simulink model "Maglev_SSC_ideal"  (R2025a)
settings: Solver=ode23t  StartTime=0.0  StopTime=T_sim  FixedStep=0.01  RelTol=1e-3  AbsTol=1e-3
PreLoadFcn:
  | modelPath = fileparts(which(bdroot));
  | run(fullfile(fileparts(modelPath), 'setup_sim_params.m'));
  | load(fullfile(fileparts(modelPath), 'Controller_Params', 'EKFData.mat'));
  | load(fullfile(fileparts(modelPath), 'Controller_Params', 'LinearControllerData.mat'));
undefined symbols (not defined in the file): Ext_Fina_Val, Ext_Init_Val, grav, I_max, I_min, mass, Plant, SSC, T_stp
libraries: fl_lib x11, nesl_utility x4
settings Model: Creator=Meng Lingbing  LastModifiedBy=CelestialAurora
settings SolverCC: AutoScaleAbsTol=off  AlgebraicLoopSolver=TrustRegion  MaxZcPerStep=1.0
settings DebuggingCC: AlgebraicLoopMsg=none  UnconnectedInputMsg=warning  UnconnectedOutputMsg=warning  UnconnectedLineMsg=warning  SymbolicDimsDataTypeCodeGenerationDiagnostic=none
settings ModelReferenceCC: EnableRefExpFcnMdlSchedulingChecks=on
settings SFSimCC: CustomCodeUndefinedFunction=UseInterfaceOnly
settings RTWCC: GPUComputeCapability=3.5  DLArmComputeVersion=19.05
settings SimscapeCC: SimscapeLogType=all  SimscapeLogSimulationStatistics=on  SimscapeLogDataHistory=10000.0

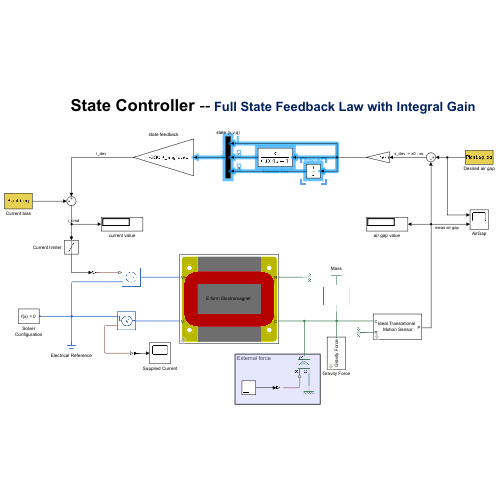
[thumbnail: Simulink's stored preview of the top-level diagram]
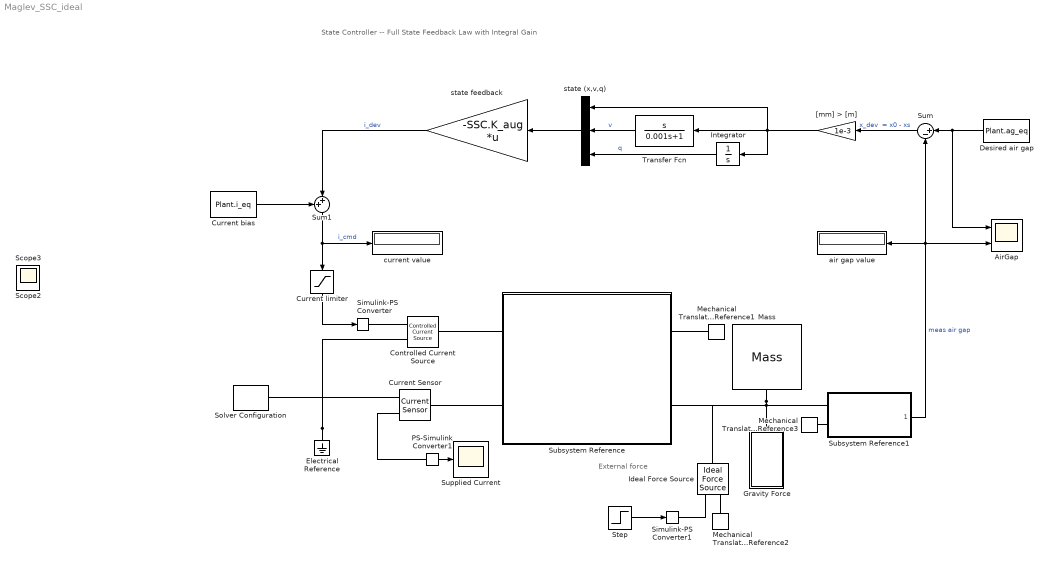
== system Maglev_SSC_ideal ==
  note: State Controller -- Full State Feedback Law with Integral Gain
  note: External force
  AirGap : Scope  NumInputPorts=2
      settings: ActiveDisplayYMinimum=0.98163587545275477  ActiveDisplayYMaximum=2.6687071249496941
  Controlled Current Source : fl_lib/Electrical/Electrical Sources/Controlled Current Source
  Current Sensor : fl_lib/Electrical/Electrical Sensors/Current Sensor
  Current bias : Constant  Value=Plant.i_eq
  Current limiter : Saturate  UpperLimit=I_max  LowerLimit=I_min
  Desired air gap : Constant  Value=Plant.ag_eq
  Electrical Reference : fl_lib/Electrical/Electrical Elements/Electrical Reference
  Gravity Force : Subsystem
      mask DialogControl DescGroupVar Prompt: Gravity Force
      mask DialogControl DescTextVar Prompt: Fg = Mass*grav, as constant parameters predefined
      mask DialogControl DescTextVar2 Prompt: Direction: Downward
      mask Display: disp("Gravity Force")
  Ideal Force Source : fl_lib/Mechanical/Mechanical Sources/Ideal Force Source
  Integrator : Integrator
  Mass : fl_lib/Mechanical/Translational Elements/Mass  mass=mass kg  num_ports=foundation.enum.numPorts2.one  v_specify=on  v_priority=Low  v=0 m/s  v_nominal_specify=off  v_nominal_value=1  v_nominal_unit=m/s  f_specify=off  f_priority=None  f=0 N  f_nominal_specify=off  f_nominal_value=700  f_nominal_unit=N
  Mechanical Translational Reference1 : fl_lib/Mechanical/Translational Elements/Mechanical Translational Reference
  Mechanical Translational Reference2 : fl_lib/Mechanical/Translational Elements/Mechanical Translational Reference
  Mechanical Translational Reference3 : fl_lib/Mechanical/Translational Elements/Mechanical Translational Reference
  PS-Simulink Converter1 : nesl_utility/PS-Simulink Converter  PhysicalDomain=network_engine_domain  SubClassName=ps_output  LeftPortType=input  RightPortType=output  PseudoPeriodic=off  Frequencies=[]  VectorFormat=inherit  Unit=inherit  AffineConversion=off
  Simulink-PS Converter : nesl_utility/Simulink-PS Converter  PhysicalDomain=network_engine_domain  SubClassName=ps_input  LeftPortType=input  RightPortType=output  PseudoPeriodic=off  Frequencies=[]  NoiseDistribution=none  NoiseParameters=[]  Unit=1  AffineConversion=off  FilteringAndDerivatives=zero  SimscapeFilterOrder=1  InputFilterTimeConstant=0.001  UdotUserProvided=0
  Simulink-PS Converter1 : nesl_utility/Simulink-PS Converter  PhysicalDomain=network_engine_domain  SubClassName=ps_input  LeftPortType=input  RightPortType=output  PseudoPeriodic=off  Frequencies=[]  NoiseDistribution=none  NoiseParameters=[]  Unit=1  AffineConversion=off  FilteringAndDerivatives=provide  SimscapeFilterOrder=1  InputFilterTimeConstant=0.001  UdotUserProvided=0
  Solver Configuration : nesl_utility/Solver Configuration  PhysicalDomain=network_engine_domain  SubClassName=solver  LeftPortType=input  RightPortType=generic  Tones=[]  Harmonics=[]  SimulateNoise=off  Profile=off  UseLocalSampling=off  EnableSwitchedLinearOptims=on  FrequencyDomain=off  UseCCode=off  RelTol=0.001  AbsTol=1e-06  MinStep=1e-09  ToWorkspace=off  RevertToSquareIcSolve=off  NumHomotopyIterations=100  PhasorMode=off  PhasorModeNumHarmonics=1  ConsistencySolver=NEWTON_XTOL_AFTER_FTOL  IndexReductionMethod=DerivativeReplacement  DoDC=off  ResidualTolerance=1e-09  ConsistencyTolSource=GLOBAL  ConsistencyAbsTol=0.001  ConsistencyRelTol=0.001  ConsistencyTolFactor=0.001  UseLocalSolver=off  LocalSolverChoice=NE_BACKWARD_EULER_ADVANCER  ResolveIndetEquations=on  FunctionEvalNumThread=1  LocalSolverSampleTime=0.001  DoFixedCost=off  MaxNonlinIter=3  MaxModeIter=2  ComputeImpulses=off  ImpulseIterations=2  LinearAlgebra=auto  LinearAlgebraNumThread=0  EquationFormulation=NE_TIME_EF  DelaysMemoryBudget=1024  AutomaticFiltering=on  FilteringTimeConstant=0.001  PartitionStorageMethod=AS_NEEDED  PartitionMemoryBudget=1024  PartitionMethod=ROBUST  MultibodyUseLocalSolver=off  MultibodyLocalSolverChoice=ODE1  MultibodyLocalSolverSampleTime=0.001
  Step : Step  Time=T_stp  Before=Ext_Init_Val  After=Ext_Fina_Val  SampleTime=0
  Subsystem Reference : Subsystem  ReferencedSubsystem=IntegratedElectromagnet  l_airgap=airgap_init
  Subsystem Reference1 : Subsystem  ReferencedSubsystem=IdealTrans_MotionSensor  ns_sw=isNoiseActive  ns_pw=NoisePower  ts=Ts  init_pos=airgap_init
  Sum : Sum  Inputs=|+-
  Sum1 : Sum  Inputs=++|
  Supplied Current : Scope
      settings: ActiveDisplayYMinimum=-2.195516974935928  ActiveDisplayYMaximum=17.297943585945966  DataLoggingVariableName=ScopeData3
  Transfer Fcn : TransferFcn  Numerator=[1 0]  Denominator=[0.001 1]
  "[mm] > [m]" : Gain  Gain=1e-3
  air gap value : Display
      settings: Decimation=4
  current value : Display
  state (x,v,q) : Mux  Inputs=3
  state feedback : Gain  Gain=-SSC.K_aug  Multiplication=Matrix(K*u) (u vector)
  Scope2 : Scope
      settings: ActiveDisplayYMinimum=2.68786  ActiveDisplayYMaximum=51.73117
  Scope3 : Scope
      settings: ActiveDisplayYMinimum=-19475.53313  ActiveDisplayYMaximum=27959.62036  DataLoggingVariableName=ScopeData2
  wires:
  state feedback/1 -> Sum1/2  "i_dev"
  Sum/1 -> "[mm] > [m]"/1  "x_dev  = x0 - xs"
  Subsystem Reference1/1 -> air gap value/1, AirGap/2, Sum/2  "meas air gap"
  Sum1/1 -> Current limiter/1, current value/1  "i_cmd"
  Desired air gap/1 -> Sum/1, AirGap/1
  Current limiter/1 -> Simulink-PS Converter/1
  Current bias/1 -> Sum1/1
  PS-Simulink Converter1/1 -> Supplied Current/1
  Integrator/1 -> state (x,v,q)/3  "q"
  state (x,v,q)/1 -> state feedback/1
  Transfer Fcn/1 -> state (x,v,q)/2  "v"
  Step/1 -> Simulink-PS Converter1/1
  "[mm] > [m]"/1 -> Transfer Fcn/1, state (x,v,q)/1, Integrator/1
  connections:
  Electrical Reference/LConn1 -- Solver Configuration/RConn1 -- Controlled Current Source/RConn2 -- Current Sensor/RConn2
  Mass/LConn1 -- Subsystem Reference1/LConn1 -- Gravity Force/RConn1 -- Subsystem Reference/RConn2 -- Ideal Force Source/LConn1
  Subsystem Reference/RConn1 -- Mechanical Translational Reference1/LConn1
  Simulink-PS Converter/RConn1 -- Controlled Current Source/RConn1
  Subsystem Reference/LConn2 -- Current Sensor/LConn1
  PS-Simulink Converter1/LConn1 -- Current Sensor/RConn1
  Subsystem Reference/LConn1 -- Controlled Current Source/LConn1
  Simulink-PS Converter1/RConn1 -- Ideal Force Source/RConn1
  Mechanical Translational Reference2/LConn1 -- Ideal Force Source/RConn2
  Mechanical Translational Reference3/LConn1 -- Subsystem Reference1/LConn2

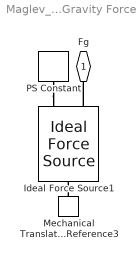
== system Maglev_SSC_ideal/Gravity Force ==
  Ideal Force Source1 : fl_lib/Mechanical/Mechanical Sources/Ideal Force Source
  Mechanical Translational Reference3 : fl_lib/Mechanical/Translational Elements/Mechanical Translational Reference
  PS Constant : fl_lib/Physical Signals/Sources/PS Constant  constant=mass*grav N
  Fg : PMIOPort  Side=Right
  connections:
  Mechanical Translational Reference3/LConn1 -- Ideal Force Source1/LConn1
  PS Constant/RConn1 -- Ideal Force Source1/RConn1
  Ideal Force Source1/RConn2 -- Fg/RConn1
